simulink model "Zalacznik_14"  (R2022a)
settings: Solver=ode5  StartTime=0.0  StopTime=20  FixedStep=0.001  RelTol=1e-3
undefined symbols (not defined in the file or in its folder): Alfa, Beta, Kd, Ki, Kp
libraries: fod x4
settings Model: Creator=Michal  LastModifiedBy=krzysiek89
settings SolverCC: AlgebraicLoopSolver=TrustRegion  AutoInsertRateTranBlk=on
settings DataIOCC: LimitDataPoints=on  SaveFormat=Array  SignalLoggingSaveFormat=ModelDataLogs  ReturnWorkspaceOutputs=off
settings OptimizationCC: ExpressionDepthLimit=2147483647  LifeSpan=inf
settings DebuggingCC: UnderspecifiedInitializationDetection=Classic  MergeDetectMultiDrivingBlocksExec=none  SolverPrmCheckMsg=warning  MultiTaskRateTransMsg=warning  FcnCallInpInsideContextMsg=warning  UnconnectedInputMsg=warning  UnconnectedOutputMsg=warning  UnconnectedLineMsg=warning  StateNameClashWarn=warning  SFUnexpectedBacktrackingDiag=warning  SFNoUnconditionalDefaultTransitionDiag=warning  SFExecutionAtInitializationDiag=none  SFMachineParentedDataDiag=warning  ArithmeticOperatorsInVariantConditions=warning
settings HardwareCC: ProdBitPerPointer=32  ProdBitPerSizeT=32  ProdBitPerPtrDiffT=32  ProdLargestAtomicFloat=None  ProdIntDivRoundTo=Undefined  ProdEndianess=Unspecified  ProdWordSize=32  ProdHWDeviceType=32-bit Generic
settings ModelReferenceCC: PropagateSignalLabelsOutOfModel=off
settings SFSimCC: SimUseLocalCustomCode=off  CustomCodeUndefinedFunction=UseInterfaceOnly
settings RTWCC: RTWUseLocalCustomCode=off
settings CodeAppCC: StateflowObjectComments=on
settings GRTTargetCC: TargetLangStandard=C89/C90 (ANSI)  CombineOutputUpdateFcns=off  GRTInterface=on
settings ConfigComp: CovMetricSettings=dw  CovSaveCumulativeToWorkspaceVar=on  CovSaveSingleToWorkspaceVar=on  CovExternalEMLEnable=off

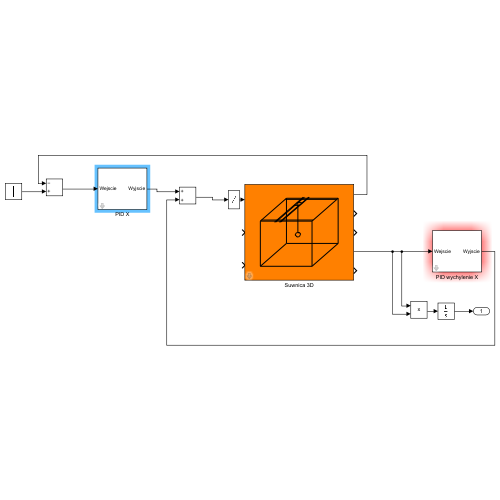
[thumbnail: Simulink's stored preview of the top-level diagram]
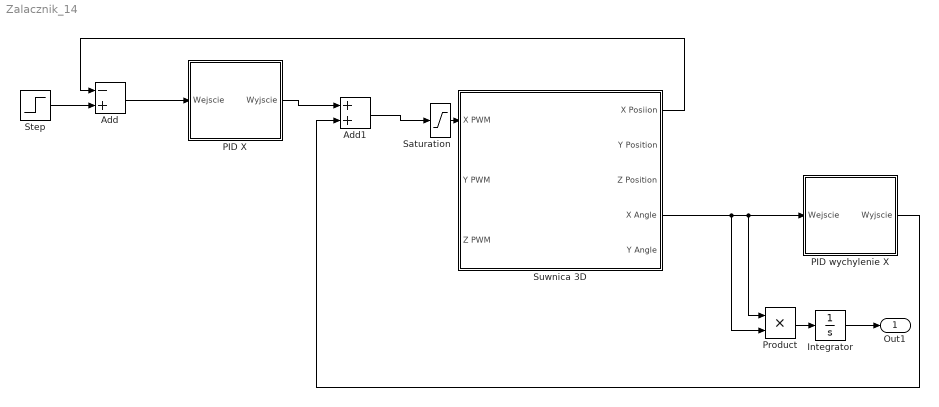
== system Zalacznik_14 ==
  Add : Sum  Inputs=-+
  Add1 : Sum
  Integrator : Integrator
  PID X : Subsystem  mask{P=41.277, I=0.007, D=6.363, Alfa=0.572, Beta=0.573}
  PID wychylenie X : Subsystem  mask{P=Kp, I=Ki, D=Kd, Alfa=Alfa, Beta=Beta}
  Product : Product
  Saturation : Saturate  UpperLimit=1  LowerLimit=-1
  Step : Step  Time=5  After=0.4  SampleTime=0
  Suwnica 3D : Subsystem  mask{RR=off, x0=[0.1, 0.1, 01,  0.01, 0.1, 0.1, 0.1, 0.1,  0.1, 0.1, -1]}
      mask prompts: RR "Model with constant length"; x0 "Initial conditions:[x,x',y,y',alfa,alfa',beta,beta',z,z',t]"
      mask Display: plot( [0 1], [0 0], [0 1], [1 1], [0 0], [0 1], [1 1], [0 1], [0.5 1.5], [0.5 0.5], [0.5 1.5], [1.5 1.5], [0.5 0.5], [0.5 1.5], [1.5 1.5], [0.5 1.5], [0 0.5], [0 0.5], [1 1.5], [0 0.5], [0 0.5], [1 1.5], [1 1.5], [1 1.5], [0.02 1.02], [1.02 1.02], [0.48 1.48], [1.48 1.48], [0.27 0.83], [0.97 1.53], [0.29 0.85], [0.97 1.53], [0.37 0.93], [0.97 1.53], [0.39 0.95], [0.97 1.53], [0.65 0.75], [1.35 1.35], [0.7 0.8], [1.4 1.4], [0.725 0.725], [1.375 0.75], 0.725+0.05*sin([0:0.5:7]), 0.7+0.05*cos([0:0.5:7]), [-0.3 -0.3], [-0.3 -0.3], [1.8 1.8], [1.8 1.8] )
  Out1 : Outport
  wires:
  Step/1 -> Add/2
  Suwnica 3D/1(X Posiion) -> Add/1
  Saturation/1 -> Suwnica 3D/1(X PWM)
  Integrator/1 -> Out1/1
  Product/1 -> Integrator/1
  Add/1 -> PID X/1(Wejscie)
  Suwnica 3D/4(X Angle) -> Product/2, Product/1, PID wychylenie X/1(Wejscie)
  Add1/1 -> Saturation/1
  PID wychylenie X/1(Wyjscie) -> Add1/2
  PID X/1(Wyjscie) -> Add1/1

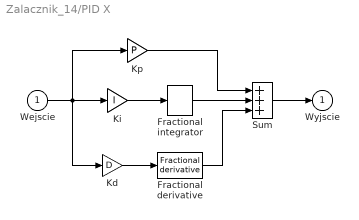
== system Zalacznik_14/PID X ==
  Wejscie : Inport
  Fractional derivative : fod/Fractional derivative  gam=Beta  ww=[0.001; 1000]  n=5  nFod=off
      settings: SourceProductName=FOMCON Toolbox
  Fractional integrator : fod/Fractional integrator  gam=Alfa  ww=[0.001; 1000]  n=5  nFod=off
      settings: SourceProductName=FOMCON Toolbox
  Kd : Gain  Gain=D  SaturateOnIntegerOverflow=on  OutDataTypeStr=Inherit: Same as input  ParamDataTypeStr=Inherit: Same as input
  Ki : Gain  Gain=I  SaturateOnIntegerOverflow=on  OutDataTypeStr=Inherit: Same as input  ParamDataTypeStr=Inherit: Same as input
  Kp : Gain  Gain=P  SaturateOnIntegerOverflow=on  OutDataTypeStr=Inherit: Same as input  ParamDataTypeStr=Inherit: Same as input
  Sum : Sum  Inputs=+++  InputSameDT=on  SaturateOnIntegerOverflow=on  OutDataTypeStr=Inherit: Same as first input
  Wyjscie : Outport  InitialOutput=0
  wires:
  Kd/1 -> Fractional derivative/1
  Wejscie/1 -> Kp/1, Ki/1, Kd/1
  Sum/1 -> Wyjscie/1
  Fractional derivative/1 -> Sum/3
  Fractional integrator/1 -> Sum/2
  Kp/1 -> Sum/1
  Ki/1 -> Fractional integrator/1

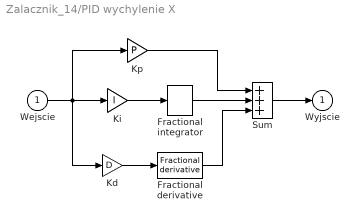
== system Zalacznik_14/PID wychylenie X ==
  Wejscie : Inport
  Fractional derivative : fod/Fractional derivative  gam=Beta  ww=[0.001; 1000]  n=5  nFod=off
      settings: SourceProductName=FOMCON Toolbox
  Fractional integrator : fod/Fractional integrator  gam=Alfa  ww=[0.001; 1000]  n=5  nFod=off
      settings: SourceProductName=FOMCON Toolbox
  Kd : Gain  Gain=D  SaturateOnIntegerOverflow=on  OutDataTypeStr=Inherit: Same as input  ParamDataTypeStr=Inherit: Same as input
  Ki : Gain  Gain=I  SaturateOnIntegerOverflow=on  OutDataTypeStr=Inherit: Same as input  ParamDataTypeStr=Inherit: Same as input
  Kp : Gain  Gain=P  SaturateOnIntegerOverflow=on  OutDataTypeStr=Inherit: Same as input  ParamDataTypeStr=Inherit: Same as input
  Sum : Sum  Inputs=+++  InputSameDT=on  SaturateOnIntegerOverflow=on  OutDataTypeStr=Inherit: Same as first input
  Wyjscie : Outport  InitialOutput=0
  wires:
  Kd/1 -> Fractional derivative/1
  Wejscie/1 -> Kp/1, Ki/1, Kd/1
  Sum/1 -> Wyjscie/1
  Fractional derivative/1 -> Sum/3
  Fractional integrator/1 -> Sum/2
  Kp/1 -> Sum/1
  Ki/1 -> Fractional integrator/1

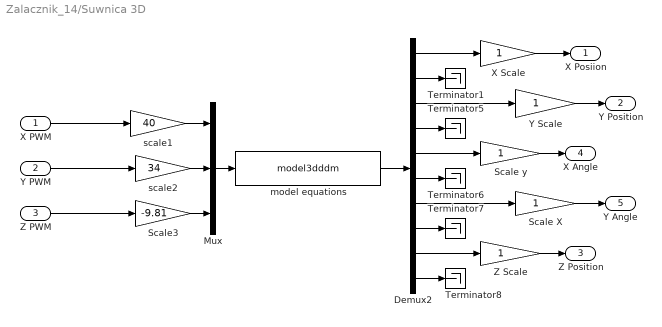
== system Zalacznik_14/Suwnica 3D ==
  X PWM : Inport
  Y PWM : Inport  Port=2
  Z PWM : Inport  Port=3
  Demux2 : Demux  Outputs=10
      settings: DisplayOption=none
  Mux : Mux  Inputs=3
  Scale X : Gain  SaturateOnIntegerOverflow=on  OutDataTypeStr=Inherit: Same as input  ParamDataTypeStr=Inherit: Same as input
  Scale y : Gain  SaturateOnIntegerOverflow=on  OutDataTypeStr=Inherit: Same as input  ParamDataTypeStr=Inherit: Same as input
  Scale3 : Gain  Gain=-9.81  SaturateOnIntegerOverflow=on  OutDataTypeStr=Inherit: Same as input  ParamDataTypeStr=Inherit: Same as input
  Terminator{1,5..8} (5 alike) : Terminator
  X Scale : Gain  SaturateOnIntegerOverflow=on  OutDataTypeStr=Inherit: Same as input  ParamDataTypeStr=Inherit: Same as input
  Y Scale : Gain  SaturateOnIntegerOverflow=on  OutDataTypeStr=Inherit: Same as input  ParamDataTypeStr=Inherit: Same as input
  Z Scale : Gain  SaturateOnIntegerOverflow=on  OutDataTypeStr=Inherit: Same as input  ParamDataTypeStr=Inherit: Same as input
  model equations : S-Function  FunctionName=model3dddm  Parameters=x0(1) x0(2) x0(3) x0(4) x0(5) x0(6) x0(7) x0(8) x0(9) x0(10) x0(11) RR  SFunctionDeploymentMode=off  EnableBusSupport=off
  scale1 : Gain  Gain=40  SaturateOnIntegerOverflow=on  OutDataTypeStr=Inherit: Same as input  ParamDataTypeStr=Inherit: Same as input
  scale2 : Gain  Gain=34  SaturateOnIntegerOverflow=on  OutDataTypeStr=Inherit: Same as input  ParamDataTypeStr=Inherit: Same as input
  X Posiion : Outport  Tag=X Position
  Y Position : Outport  Port=2
  Z Position : Outport  Port=3
  X Angle : Outport  Port=4
  Y Angle : Outport  Port=5
  wires:
  Mux/1 -> model equations/1
  Y Scale/1 -> Y Position/1
  model equations/1 -> Demux2/1
  X Scale/1 -> X Posiion/1
  Demux2/1 -> X Scale/1
  Demux2/3 -> Y Scale/1
  Z Scale/1 -> Z Position/1
  Demux2/9 -> Z Scale/1
  Scale y/1 -> X Angle/1
  Demux2/5 -> Scale y/1
  Scale X/1 -> Y Angle/1
  Demux2/7 -> Scale X/1
  Demux2/2 -> Terminator1/1
  Demux2/4 -> Terminator5/1
  Demux2/6 -> Terminator6/1
  Demux2/8 -> Terminator7/1
  Demux2/10 -> Terminator8/1
  scale2/1 -> Mux/2
  Y PWM/1 -> scale2/1
  Scale3/1 -> Mux/3
  Z PWM/1 -> Scale3/1
  scale1/1 -> Mux/1
  X PWM/1 -> scale1/1
